simulink model "delay_without_delay_block"  (R2018b)
settings: Solver=FixedStepDiscrete  StartTime=0.0  StopTime=10.0  RelTol=1e-3
libraries: simulink x2
settings Model: DataTypeOverride=Double  MinMaxOverflowLogging=ForceOff  Creator=marwan  LastModifiedBy=marwan

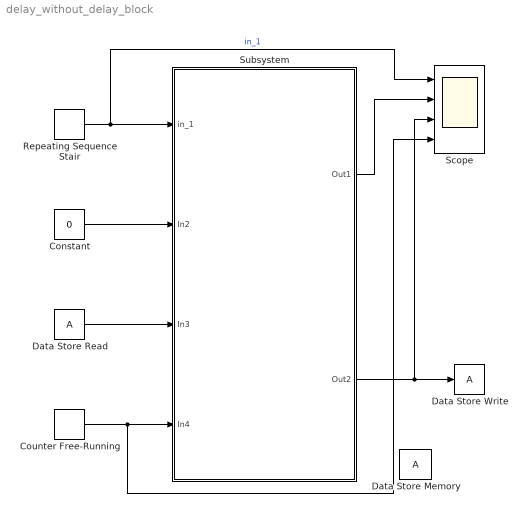
== system delay_without_delay_block ==
  Constant : Constant  Value=0
  Counter Free-Running : simulink/Sources/Counter Free-Running  NumBits=3  tsamp=-1
  Data Store Memory : DataStoreMemory  ReadBeforeWriteMsg=warning  WriteAfterWriteMsg=warning  WriteAfterReadMsg=warning  ShowAdditionalParam=off
  Data Store Read : DataStoreRead
  Data Store Write : DataStoreWrite
  Repeating Sequence Stair : simulink/Sources/Repeating Sequence Stair  OutValues=[3 5 2 4 1 6 7 5]  tsamp=-1  OutMin=[]  OutMax=[]  OutDataTypeStr=double  OutputDataTypeScalingMode=double  OutDataType=fixdt(0,8)  ConRadixGroup=Best Precision: Vector-wise  OutScaling=2^-12
  Scope : Scope  NumInputPorts=4
  Subsystem : Subsystem
  wires:
  Repeating Sequence Stair/1 -> Subsystem/1(in_1), Scope/1  "in_1"
  Counter Free-Running/1 -> Subsystem/4(In4), Scope/4
  Subsystem/2(Out2) -> Scope/3, Data Store Write/1
  Constant/1 -> Subsystem/2(In2)
  Data Store Read/1 -> Subsystem/3(In3)
  Subsystem/1(Out1) -> Scope/2

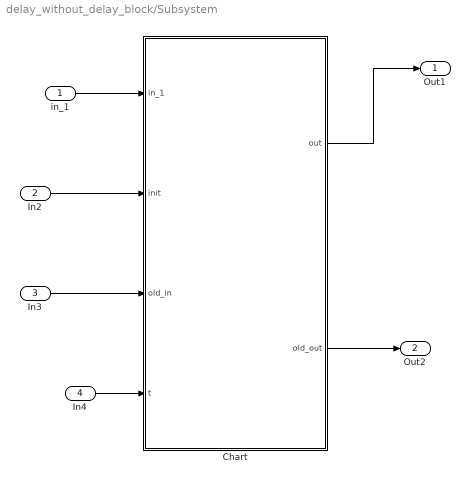
== system delay_without_delay_block/Subsystem ==
  in_1 : Inport
  In2 : Inport  Port=2
  In3 : Inport  Port=3
  In4 : Inport  Port=4
  Chart : Stateflow chart  TreatAsAtomicUnit=on
  Out1 : Outport
  Out2 : Outport  Port=2
  wires:
  In3/1 -> Chart/3(old_in)
  Chart/2(old_out) -> Out2/1
  in_1/1 -> Chart/1(in_1)
  In4/1 -> Chart/4(t)
  Chart/1(out) -> Out1/1
  In2/1 -> Chart/2(init)

== stateflow chart delay_without_delay_block/Subsystem/Chart ==
  (default) -> (junction 13)
  (junction 13) -> (junction 14) [order 1] : [t==1]
  (junction 13) -> (junction 15) [order 2] : {out=old_in;
      | old_out=in_1;}
  (junction 14) -> (junction 16) : {out=init;
      | old_out=in_1;}
  (junction 16) -> (junction 15)
  (junction 15) -> (junction 17)
  data: in_1 input; init input; old_in input; out output; old_out output; t input
